simulink model "LR_3_var15_5"  (R2020b)
settings: Solver=ode3  StartTime=0.0  StopTime=2  FixedStep=1e-3  RelTol=1e-3
libraries: simulink x1
settings Model: Creator=SIA  LastModifiedBy=SIA

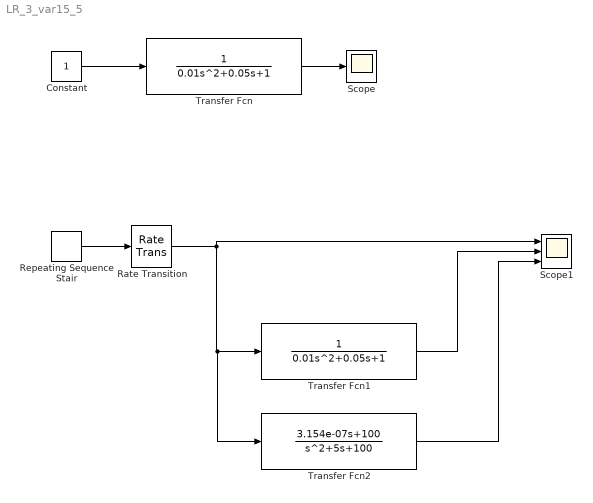
== system LR_3_var15_5 ==
  Constant : Constant
  Rate Transition : RateTransition  OutPortSampleTime=1e-3
  Repeating Sequence Stair : simulink/Sources/Repeating Sequence Stair  OutValues=[3 1 1 1 4 2 2 2 1 0 -1 2 4 1 2 2].'  tsamp=0.05  OutMin=[]  OutMax=[]  OutDataTypeStr=double  OutputDataTypeScalingMode=double  OutDataType=fixdt(0,8)  ConRadixGroup=Best Precision: Vector-wise  OutScaling=2^-12
  Scope : Scope
  Scope1 : Scope  NumInputPorts=3
  Transfer Fcn : TransferFcn  Denominator=[0.01 0.05 1]
  Transfer Fcn1 : TransferFcn  Denominator=[0.01 0.05 1]
  Transfer Fcn2 : TransferFcn  Numerator=[3.154e-07 100]  Denominator=[1 5 100]
  wires:
  Constant/1 -> Transfer Fcn/1
  Transfer Fcn/1 -> Scope/1
  Repeating Sequence Stair/1 -> Rate Transition/1
  Rate Transition/1 -> Scope1/1, Transfer Fcn2/1, Transfer Fcn1/1
  Transfer Fcn1/1 -> Scope1/2
  Transfer Fcn2/1 -> Scope1/3
